simulink model "PSC_Full_2026_02_11"  (R2024b)
settings: Solver=VariableStepAuto  StartTime=0.0  StopTime=1  RelTol=1e-3
libraries: spsControlledVoltageSourceLib x1, spsCurrentMeasurementLib x1, spsPVArrayLib x1, simulink x1, spsVoltageMeasurementLib x1, sps_lib x1
settings Model: Creator=kimiaahmadi  LastModifiedBy=kimiaahmadi

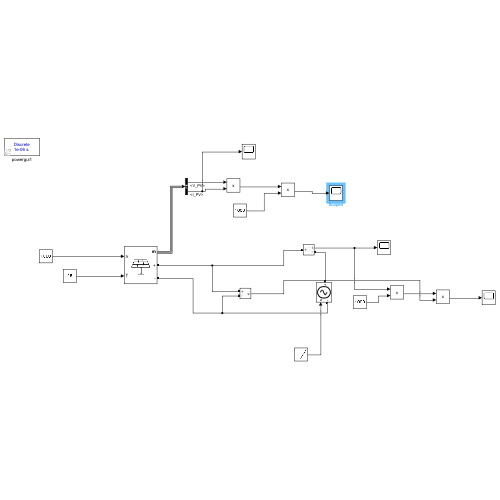
[thumbnail: Simulink's stored preview of the top-level diagram]
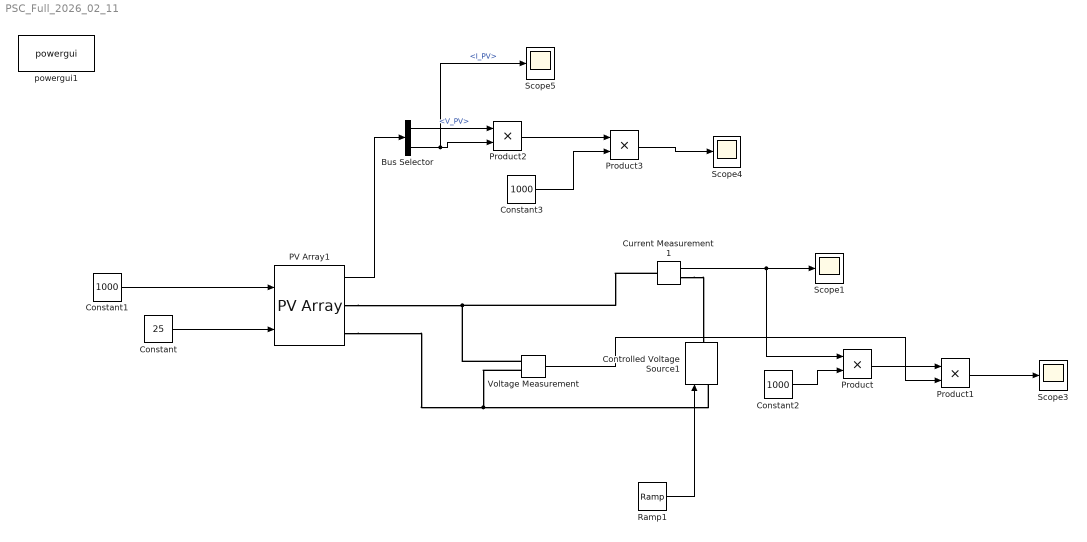
== system PSC_Full_2026_02_11 ==
  Bus Selector : BusSelector  OutputSignals=V_PV,I_PV
  Constant : Constant  Value=25
  Constant1 : Constant  Value=1000
  Constant2 : Constant  Value=1000
  Constant3 : Constant  Value=1000
  Controlled Voltage Source1 : spsControlledVoltageSourceLib/Controlled Voltage Source  Initialize=on  Source_Type=AC  Amplitude=0  Phase=0  Frequency=0  Measurements=None
  Current Measurement1 : spsCurrentMeasurementLib/Current Measurement  PhasorSimulation=off  OutputType=Complex  PSBequivalent=0
  PV Array1 : spsPVArrayLib/PV Array  Npar=1  Nser=1  PlotType=array @ 25 deg.C & specified irradiances  S_vec="[ 1000  500    400  300]"  Temp_C_vec="[ 45 25  ]"  ModuleName=User-defined  PlotWhenSelected=off  Pm=0.25  Ncell=1  Voc=0.60754  Isc=0.5737715  Vm=0.47  Im=0.53191489  beta_Voc_pc=-0.36099  alpha_Isc_pc=0.102  beta_Voc=-0.0021932  alpha_Isc=0.00058525  IL=0.57515  I0=2.136e-11  nI=0.98547  Rsh=51.3567  Rs=0.12324  RobustModel=off  RobustCellTemperature=313.3991  BAL=off  Tc=1e-6  Tfilter=5e-5
  Product{,1..3} (4 alike) : Product
  Ramp1 : simulink/Sources/Ramp  slope=1  start=0  InitialOutput=0
  Scope{1,3..5} (4 alike) : Scope
  Voltage Measurement : spsVoltageMeasurementLib/Voltage Measurement  PhasorSimulation=off  OutputType=Complex  PSBequivalent=0
  powergui1 : sps_lib/powergui  Priority=1  SimulationMode=Discrete  SampleTime=1e-6  frequency=60  Iterations=50  frequencyindice=0  Pbase=100e6  ErrMax=1e-4  UnitsV=kV  UnitsW=MW  buscounter=0  FunctionMessages=off  echomessages=off  EnableUseOfTLC=off  CurrentSourceSwitches=off  DisableSnubberDevices=off  DisableRonSwitches=off  DisableVfSwitches=off  DisplayEquations=off  AutomaticDiscreteSolvers=off  SolverType=Tustin/Backward Euler (TBE)  Interpol=off  ExternalGateDelay=off  methode=off  Ts=100  x0status=blocks  SPID=on  SwTol=0  HookPort=off  NonlinearTolerance=1e-4  nMaxIteration=100  ContinueOnMaxIteration=off  RestoreLinks=warning  ResistiveCurrentMeasurement=off  Frange=[0:2:500]  Ylog=off  Xlog=on  ShowGrid=off  save=off  variable=ZData  structure=0  ZoomFFT=off  StartTime=0.0  cycles=1  DisplayStyle=1  fundamental=60  FreqAxis=off  MaxFrequency=1000  frequencyindicesteady=1  RmsSteady=1  display=off
  wires:
  Voltage Measurement/1 -> Product1/2
  Product2/1 -> Product3/1
  Constant3/1 -> Product3/2
  Product/1 -> Product1/1
  Product1/1 -> Scope3/1
  Ramp1/1 -> Controlled Voltage Source1/1
  Constant1/1 -> PV Array1/1
  PV Array1/1 -> Bus Selector/1
  Constant2/1 -> Product/2
  Product3/1 -> Scope4/1
  Current Measurement1/1 -> Product/1, Scope1/1
  Constant/1 -> PV Array1/2
  Bus Selector/2 -> Scope5/1, Product2/2  "<I_PV>"
  Bus Selector/1 -> Product2/1  "<V_PV>"
  connections:
  Voltage Measurement/LConn1 -- PV Array1/RConn1 -- Current Measurement1/LConn1
  Controlled Voltage Source1/LConn1 -- PV Array1/RConn2 -- Voltage Measurement/LConn2
  Current Measurement1/RConn1 -- Controlled Voltage Source1/RConn1
